simulink model "Chua_LQr"  (R2014b)
settings: Solver=ode45  StartTime=0.0  StopTime=20  FixedStep=0.025  RelTol=1e-6
values from neighbouring files (symbols this model uses):
  x0 = [0.2;0.1;-0.3;0.3;0.5;-0.2]    [Main_ChuaLQR.m]
undefined symbols (not defined in the file or in its folder): K
settings Model: Creator=gianni  LastModifiedBy=gianni

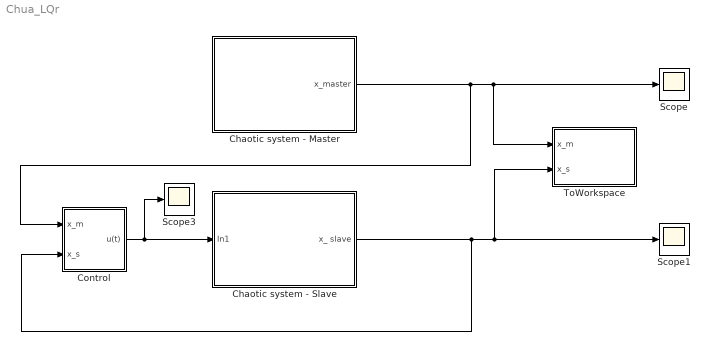
== system Chua_LQr ==
  Chaotic system - Master : Subsystem
  Chaotic system - Slave : Subsystem
  Control : Subsystem
  Scope : Scope
  Scope1 : Scope
      settings: YMin=-1e+08  YMax=3e+08
  Scope3 : Scope
      settings: SaveName=ScopeData3
  ToWorkspace : Subsystem
  wires:
  Control/1(u(t)) -> Scope3/1, Chaotic system - Slave/1(In1)
  Chaotic system - Master/1(x_master) -> Control/1(x_m), ToWorkspace/1(x_m), Scope/1
  Chaotic system - Slave/1(x_ slave) -> Control/2(x_s), ToWorkspace/2(x_s), Scope1/1

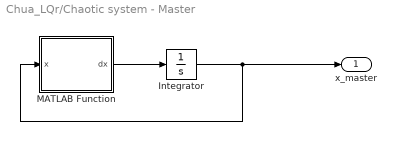
== system Chua_LQr/Chaotic system - Master ==
  Integrator : Integrator  InitialCondition=x0([1:3])
  MATLAB Function : MATLAB Function  TreatAsAtomicUnit=on
  x_master : Outport
  wires:
  MATLAB Function/1(dx) -> Integrator/1
  Integrator/1 -> x_master/1, MATLAB Function/1(x)

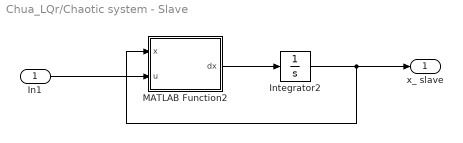
== system Chua_LQr/Chaotic system - Slave ==
  In1 : Inport
  Integrator2 : Integrator  InitialCondition=x0([4:6])
  MATLAB Function2 : MATLAB Function  TreatAsAtomicUnit=on
  x_ slave : Outport
  wires:
  MATLAB Function2/1(dx) -> Integrator2/1
  Integrator2/1 -> x_ slave/1, MATLAB Function2/1(x)
  In1/1 -> MATLAB Function2/2(u)

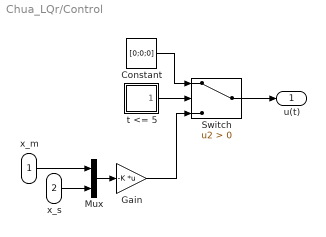
== system Chua_LQr/Control ==
  x_m : Inport
  x_s : Inport  Port=2
  Constant : Constant  Value=[0;0;0]
  Gain : Gain  Gain=-K  Multiplication=Matrix(K*u)
  Mux : Mux  Inputs=2
  Switch : Switch  Criteria=u2 > Threshold
  t <= 5 : Subsystem
  u(t) : Outport
  wires:
  Gain/1 -> Switch/3
  x_s/1 -> Mux/2
  x_m/1 -> Mux/1
  Mux/1 -> Gain/1
  t <= 5/1(t <= 5) -> Switch/2
  Constant/1 -> Switch/1
  Switch/1 -> u(t)/1

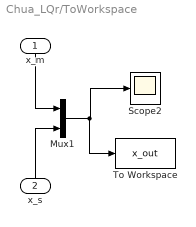
== system Chua_LQr/ToWorkspace ==
  x_m : Inport
  x_s : Inport  Port=2
  Mux1 : Mux  Inputs=2
  Scope2 : Scope
      settings: SaveName=ScopeData2
  To Workspace : ToWorkspace  VariableName=x_out  SaveFormat=Timeseries  SampleTime=-1
  wires:
  Mux1/1 -> To Workspace/1, Scope2/1
  x_s/1 -> Mux1/2
  x_m/1 -> Mux1/1

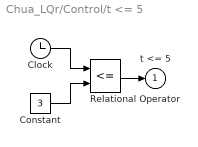
== system Chua_LQr/Control/t <= 5 ==
  Clock : Clock
  Constant : Constant  Value=3
  Relational Operator : RelationalOperator  Operator=<=  InputSameDT=on
  t <= 5 : Outport  InitialOutput=0
  wires:
  Constant/1 -> Relational Operator/2
  Clock/1 -> Relational Operator/1
  Relational Operator/1 -> t <= 5/1

== matlab function Chua_LQr/Chaotic system - Master/MATLAB Function ==
  data: x input; dx output
function dx = ode(x)                             
    p = 10;q = 100/7;                             % Parameters                 
    x1 = x(1);y1 = x(2);z1 = x(3);
    
    f_x1 = 2*x1^3 - x1/7;
    
    dx = [p*(y1-f_x1);
          x1-y1+z1;
          -q*y1;          
          ];  
end

== matlab function Chua_LQr/Chaotic system - Slave/MATLAB Function2 ==
  data: x input; dx output; u input
function dx = ode(x,u)                             
    p = 10;q = 100/7;                             % Parameters                 
    x1 = x(1);y1 = x(2);z1 = x(3);
    ux = u(1);uy = u(2); uz = u(3);
    
    f_x1 = 2*x1^3 - x1/7;
    
    dx = [p*(y1-f_x1) + ux;
          x1-y1+z1 + uy;
          -q*y1 + uz;          
          ];  
end
